simulink model "mdaq_adc"  (R2013a)
settings: Solver=FixedStepDiscrete  StartTime=0.0  StopTime=10.0  RelTol=1e-3
libraries: microdaq_lib x1
settings Model: Creator=peselnikmg  LastModifiedBy=peselnikmg
settings DataIOCC: SignalLoggingSaveFormat=ModelDataLogs  SaveOutput=off  SignalLogging=off  DSMLogging=off  SaveTime=off
settings OptimizationCC: InlineParams=on  EnhancedBackFolding=on  OptimizeModelRefInitCode=on  LifeSpan=1
settings HardwareCC: ProdBitPerLong=40  ProdLargestAtomicInteger=Integer  ProdIntDivRoundTo=Zero  ProdEndianess=LittleEndian  ProdHWDeviceType=Texas Instruments->C6000
settings RTWCC: SystemTargetFile=microdaq.tlc  TemplateMakefile=microdaq.tmf  PostCodeGenCommand=microdaq_postcodegen(buildInfo)  Description=MicroDAQ Real-Time Measurement System  GenerateReport=on  ProcessScript=microdaq_make_rtw_hook  IncludeHyperlinkInReport=on
settings CodeAppCC: IgnoreCustomStorageClasses=off
settings STFCustomTargetCC: CodeReplacementLibrary=TI C674x  IncludeMdlTerminateFcn=off  CombineOutputUpdateFcns=on  SuppressErrorStatus=on  ERTCustomFileBanners=on  SupportAbsoluteTime=off  SupportNonFinite=off  SupportComplex=off  SupportContinuousTime=off  SupportNonInlinedSFcns=off  MATLABClassNameForMDSCustomization=Simulink.SoftwareTarget.ERTCustomization  SystemTargetFile=microdaq.tlc
settings ERTTargetCC: CodeReplacementLibrary=TI C674x  GenerateSampleERTMain=off  ParMdlRefBuildCompliant=off  CompOptLevelCompliant=off  ConcurrentExecutionCompliant=off  IncludeMdlTerminateFcn=off  SuppressErrorStatus=on  ERTFirstTimeCompliant=off  SupportAbsoluteTime=off  SupportNonFinite=off  SupportComplex=off  ModelStepFunctionPrototypeControlCompliant=off  CPPClassGenCompliant=off  ERTCustomFileTemplate=microdaq_main.tlc

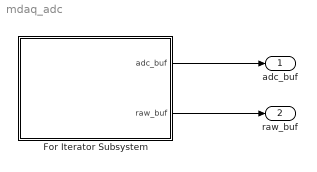
== system mdaq_adc ==
  For Iterator Subsystem : Subsystem  TreatAsAtomicUnit=on  mask{BufSize=100}
      mask prompts: BufSize "Buffer size:"
      mask Display: fprintf('Buffer size: %d\n',BufSize);
  adc_buf : Outport  SampleTime=0.1
  raw_buf : Outport  Port=2  SampleTime=0.1
  wires:
  For Iterator Subsystem/1(adc_buf) -> adc_buf/1
  For Iterator Subsystem/2(raw_buf) -> raw_buf/1

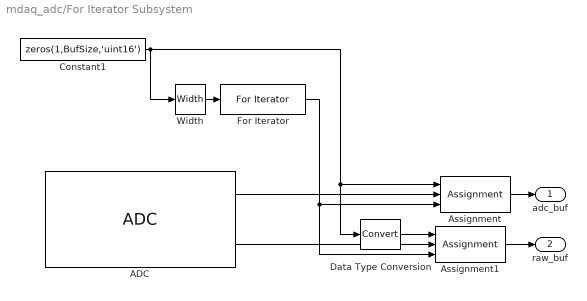
== system mdaq_adc/For Iterator Subsystem ==
  ADC : microdaq_lib/ADC  Channel=1  pPolarity=Bipolar  pRange=10V  pMode=Single-ended  SampleTime=-1
  Assignment : Assignment  IndexOptions=Index vector (port)  Indices=1  OutputSizes=100
  Assignment1 : Assignment  IndexOptions=Index vector (port)  Indices=1  OutputSizes=100
  Constant1 : Constant  Value=zeros(1,BufSize,'uint16')
  Data Type Conversion : DataTypeConversion
  For Iterator : ForIterator  IterationSource=external  IterationLimit=100
  Width : Width
  adc_buf : Outport
  raw_buf : Outport  Port=2
  wires:
  ADC/1 -> Assignment/2
  Assignment/1 -> adc_buf/1
  For Iterator/1 -> Assignment1/3, Assignment/3
  Constant1/1 -> Width/1, Data Type Conversion/1, Assignment/1
  Width/1 -> For Iterator/1
  Assignment1/1 -> raw_buf/1
  ADC/2 -> Assignment1/2
  Data Type Conversion/1 -> Assignment1/1
